simulink model "cvtModel"  (R2019a)
settings: Solver=VariableStepAuto  StartTime=0.0  StopTime=80  FixedStep=1e-3  RelTol=1e-3  AbsTol=1e-3  EnableMultiTasking=on
PreLoadFcn:
  | m1=3.5;
  | m2=3.2;
  | mr1=0.8;
  | mr2=0.7;
  | speedVector=[1508.85099817596;1518.45723596462;1530.44196592720;1537.65262467286;1544.87011816615;1563.98348990289;1583.08660951818;1616.48460379372;1668.91395283447;1709.42350201510;1752.30812599583;1799.96340381967;1847.59134265301;1904.74008492967;1971.45405650923;2028.61646828115;2083.40038787914;2140.55254752961;2190.54189166781;2259.62068592604;2323.95274795787;2376.37867962481;2443.06531221387;2519.28983511532;2576.50350749443;2612.24923757958;2650.37004246484;2681.37245769738;2717.13869202541;2771.92602899721;2819.56080257817;2855.26894155137;2890.95315890788;2938.61868885316;2976.76341535511;2991.07537688442;3019.63778721441;3045.79436637996;3071.94069342408;3093.34370561560;3114.80823053575;3141.04340929901;3172.04240715774;3186.35436868705;3214.89627477416;3231.51496362732;3267.18209411476;3333.83797033950;3371.93485360807;3421.93444986770;3488.60057821388;3540.98550139507;3586.19052219491;3617.10408570831;3674.22548899447;3712.24719003915;3731.22044944954;3740.69340965949;3759.66325169607;3771.50786933232;3785.72414439486;3792.79810818800;3797.48674505959;3802.17879930499;3806.87085355039;3816.26521416264;3820.89917305322;3827.93896310823;3835.00950952755;3839.71865064202];
  | torqueVector=[15.4893802008608;16.0795925394548;16.6441434720229;17.1317101865136;17.6705997130559;18.1068436154950;18.4661032998565;18.8510243902439;19.0563156384505;19.1846226685796;19.2616068866571;19.3899139167862;19.3129296987087;19.1846226685796;19.3385911047346;19.3129296987087;19.3129296987087;19.2102840746054;18.9793314203730;19.0049928263988;19.1589612625538;19.3385911047346;19.2872682926829;19.3129296987087;19.6721893830703;19.8004964131994;19.8774806312769;20.1597560975610;20.4420315638450;20.4676929698709;20.4420315638450;20.2880631276901;19.9544648493544;20.1597560975610;20.4163701578192;20.5703385939742;20.4163701578192;20.0827718794835;19.6721893830703;19.4155753228120;19.6208665710186;19.8774806312769;20.1340946915351;20.2880631276901;19.9801262553802;19.5695437589670;19.1076384505021;18.8253629842181;18.7227173601148;18.5687489239598;18.3634576757532;18.2351506456241;17.8502295552367;17.4653084648493;17.1317101865136;16.4645136298422;15.8486398852224;15.4380573888092;14.7965222381636;14.3089555236729;13.7444045911047;13.2055150645624;12.6409641319943;12.1020746054519;11.5631850789096;10.5623902439024;9.58725681492108;8.79175322812051;8.22720229555236;7.81661979913916];
model workspace (MAT data in the model file):
  DOWN_TABLE = [0  5  20  35; 0  5  20  35; 0  5  25  40; 0  5  30  50; 0  30  50  80; 0  30  50  80]
  DOWN_TH_BP = [0; 0.05; 0.4; 0.5; 0.9; 1]
  TWAIT = 2
  UP_TABLE = [10  30  50  1000000; 10  30  50  1000000; 15  30  50  1000000; 23  41  60  1000000; 40  70  100  1000000; 40  70  100  1000000]
  UP_TH_BP = [0; 0.25; 0.35; 0.5; 0.9; 1]
  clutchRise = 0.1
  eff_tor_rad = 0.4
  engagement_area = 0.0025
  fric_coeff = 0.5
  num_fric_surf = 6
  p0 = 2000000
  peak_normal = 0.55
  pressThresh = 0.05
  velTol = 0.001
undefined symbols (not defined in the file): sigbuilder_block
libraries: fl_lib x21, sdl_lib x9, nesl_utility x8
CloseFcn:
  | try,close(h1_sdl_car),end
  | clear h1_sdl_car
  | 
  | clear simlog_sdl_car
  | clear logsout_sdl_car
Description:
  | Vehicle with Four-Speed Transmission
  | 
  | Copyright 2008-2016 The MathWorks, Inc.
settings Model: FPTRunName=Active  PacingRate=5  ExtModeAutoUpdateStatusClock=off  Creator=MathWorks
settings SolverCC: AutoScaleAbsTol=off  ZcThreshold=0  ZeroCrossAlgorithm=Adaptive
settings DataIOCC: LimitDataPoints=on  MaxDataPoints=10000  SaveOutput=off  DSMLogging=off  SaveTime=off  ReturnWorkspaceOutputs=off  SignalLoggingName=logsout_cvtModel
settings OptimizationCC: ExpressionDepthLimit=2147483647  InitFltsAndDblsToZero=on  LifeSpan=inf
settings DebuggingCC: AlgebraicLoopMsg=none  SaveWithParameterizedLinksMsg=none  UnderspecifiedInitializationDetection=Classic  MergeDetectMultiDrivingBlocksExec=none  CheckExecutionContextPreStartOutputMsg=on  SignalResolutionControl=TryResolveAllWithWarning  MaskedZcDiagnostic=none  MultiTaskDSMMsg=warning  MultiTaskCondExecSysMsg=none  SigSpecEnsureSampleTimeMsg=none  FcnCallInpInsideContextMsg=warning  AllowSymbolicDim=off  StateNameClashWarn=warning  SFUnexpectedBacktrackingDiag=warning  SFNoUnconditionalDefaultTransitionDiag=warning  SFExecutionAtInitializationDiag=none  ArithmeticOperatorsInVariantConditions=warning
settings HardwareCC: ProdBitPerPointer=32  ProdBitPerSizeT=32  ProdBitPerPtrDiffT=32  ProdLargestAtomicFloat=None  ProdIntDivRoundTo=Undefined  ProdEndianess=Unspecified  ProdWordSize=32  ProdHWDeviceType=32-bit Generic  TargetBitPerLong=64  TargetBitPerPointer=64  TargetBitPerSizeT=64  TargetBitPerPtrDiffT=64  TargetLongLongMode=on  TargetIntDivRoundTo=Zero  TargetEndianess=LittleEndian  TargetWordSize=64  TargetHWDeviceType=MATLAB Host  ProdEqTarget=off
settings ModelReferenceCC: UpdateModelReferenceTargets=IfOutOfDate  PropagateSignalLabelsOutOfModel=off
settings SFSimCC: SimUseLocalCustomCode=off
settings RTWCC: Description=Generic Real-Time Target  RTWUseLocalCustomCode=off
settings CodeAppCC: StateflowObjectComments=on
settings GRTTargetCC: TargetLangStandard=C89/C90 (ANSI)  CombineOutputUpdateFcns=off  GRTInterface=on
settings ConfigComp: CovMetricSettings=dw  CovSaveCumulativeToWorkspaceVar=on  CovSaveSingleToWorkspaceVar=on  CovExternalEMLEnable=off  CovBoundaryAbsTol=1.0e-5
settings SimscapeCC: SimscapeNormalizeSystem=off  SimscapeLogType=all  SimscapeLogSimulationStatistics=on

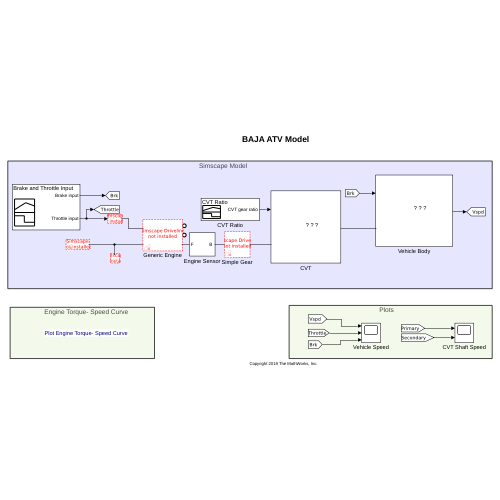
[thumbnail: Simulink's stored preview of the top-level diagram]
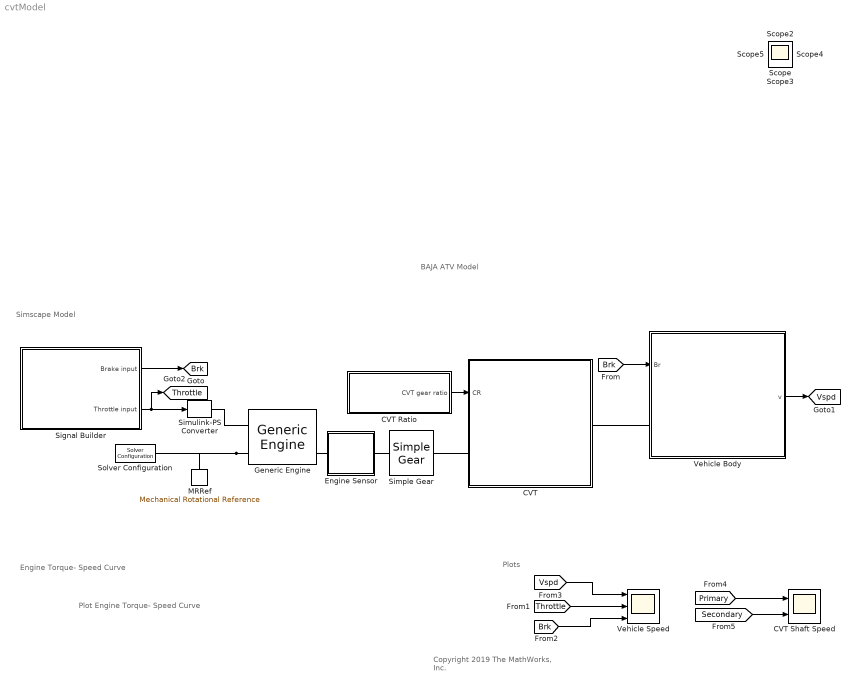
== system cvtModel ==
  note: Simscape Model
  note: Plots
  note: BAJA ATV Model
  note: Copyright 2019 The MathWorks, Inc.
  note: Plot Engine Torque- Speed Curve
  note: Engine Torque- Speed Curve
  CVT : Subsystem
      mask Display: image("CVT.jpg")
  CVT Ratio : Subsystem  Tag=STV Subsys  LoadFcn=sigbuilder_block('load');  StartFcn=sigbuilder_block('start');  StopFcn=sigbuilder_block('stop');  ClipboardFcn=sigbuilder_block('clipboard');  mask(Sigbuilder block){tuvar=[0:10]}
      mask help: Simulink:masks:SigbuilderBlock_MD
      mask init:
      | if ~strcmp(get_param(bdroot(gcbh),'SimulationStatus'),'stopped') tuvar = sigbuilder_block('maskInit'); end
      settings: CopyFcn=sigbuilder_block('copy');  DeleteFcn=sigbuilder_block('delete');  ModelCloseFcn=sigbuilder_block('modelClose');  PreSaveFcn=sigbuilder_block('preSave');  PauseFcn=sigbuilder_block('pause');  ContinueFcn=sigbuilder_block('continue');  NameChangeFcn=sigbuilder_block('namechange');  OpenFcn=sigbuilder_block('open',[6 61.5 948 414.75 ]);  CloseFcn=sigbuilder_block('close');
      mask Display: plot(0, 0, 100, 100,[2, 2, 32, 32, 2], [68, 8, 8, 68, 68],[32, 2], [38, 38], [32, 19, 2],[53, 60, 44], [32, 17, 17, 2],[16, 16, 31, 31]);txt = getActiveGroup(gcbh);text(2, 100, txt,'verticalAlignment', 'top');
  CVT Shaft Speed : Scope  NumInputPorts=2
  Engine Sensor : Subsystem
  Generic Engine : sdl_lib/Engines/Generic Engine  model_parameterization=2  engine_type=1  P_max=100 kW  w_P_max=4500 rpm  w_max=5000 rpm  w_min=500 rpm  w_tab=speedVector rpm  trq_tab=torqueVector N*m  pwr_tab=[20, 40, 78, 120, 145, 148, 125, 60] kW  interp_method=simscape.enum.interpolation.linear  model_inertia=1  inertia=1 kg*m^2  initial_velocity=2100 rpm  model_time_constant=0  time_constant=0.4 s  T0=0  w_thr=100 rpm  idle_speed=0  idle_speed_reference=2500 rpm  tau_controller=1 s  idle_w_thr=1 rpm  redline=0  redline_speed=5000 rpm  tau_redline=1 s  redline_w_thr=1 rpm  fc_model=0  fc_per_rev=25 mg/rev  displaced_volume=400 cm^3  rev_per_cycle=2  fc_w_tab=[1000, 2000, 3000, 4000, 5000, 6000] rpm  fc_trq_tab=[0, 80, 160, 200, 240, 320, 360, 400] N*m  fc_tab=[.5, .9, 1.4, 1.6, 1.9, 2.7, 3.4, 4.4; 1, 1.7, 2.7, 3.1, 3.6, 5, 6, 7.4; 1.4, 2.7, 4, 4.8, 5.6, 7.5, 8.5, 10.5; 2, 3.6, 5.8, 6.7, 8, 10.4, 11.7, 13.3; 2.5, 4.8, 7.9, 9.4, 10.8, 14, 16.2, 18.6; 3.1, 6, 10.3, 11.9, 13.8, 18.4, 22, 26.5] g/s  bmep_tab=[0, 250, 500, 625, 750, 1000, 1150, 1250] kPa  bsfc_tab=[410, 380, 300, 280, 270, 290, 320, 380; 410, 370, 290, 270, 260, 270, 285, 320; 415, 380, 290, 275, 265, 270, 270, 300; 420, 390, 310, 290, 285, 280, 280, 285; 430, 410, 340, 320, 310, 300, 310, 320; 450, 430, 370, 340, 330, 330, 350, 380] g/hr/kW  fc_interp_method=simscape.enum.interpolation.linear
      settings: SourceProductName=Simscape Driveline
  MRRef : fl_lib/Mechanical/Rotational Elements/Mechanical Rotational Reference
  Signal Builder : Subsystem  Tag=STV Subsys  LoadFcn=sigbuilder_block('load');  StartFcn=sigbuilder_block('start');  StopFcn=sigbuilder_block('stop');  ClipboardFcn=sigbuilder_block('clipboard');  mask(Sigbuilder block){tuvar=[0:10]}
      mask help: Simulink:masks:SigbuilderBlock_MD
      mask init:
      | if ~strcmp(get_param(bdroot(gcbh),'SimulationStatus'),'stopped') tuvar = sigbuilder_block('maskInit'); end
      settings: CopyFcn=sigbuilder_block('copy');  DeleteFcn=sigbuilder_block('delete');  ModelCloseFcn=sigbuilder_block('modelClose');  PreSaveFcn=sigbuilder_block('preSave');  PauseFcn=sigbuilder_block('pause');  ContinueFcn=sigbuilder_block('continue');  NameChangeFcn=sigbuilder_block('namechange');  OpenFcn=sigbuilder_block('open',[235.5 66.5 481 367 ]);  CloseFcn=sigbuilder_block('close');
      mask Display: plot(0, 0, 100, 100,[2, 2, 32, 32, 2], [68, 8, 8, 68, 68],[32, 2], [38, 38], [32, 19, 2],[53, 60, 44], [32, 17, 17, 2],[16, 16, 31, 31]);txt = getActiveGroup(gcbh);text(2, 100, txt,'verticalAlignment', 'top');
  Simple Gear : sdl_lib/Gears/Simple Gear  ratio=4  rotation_direction=1  friction_model=1  T_noload=0.1 N*m  T_nom=5 N*m  efficiency_nom=0.8  efficiency=0.8  mu_visc=[0, 0] N*m/(rad/s)  w_thr=0.01 rad/s  pwr_thr=0.001 W  enable_faults=0  efficiency_fault=0.05  external_fault=simscape.enum.onoff.off  temporal_fault=0  fault_time=5 s  fault_angles=pi / 12 rad  report_fault=1  temperature_TLU=[280, 300, 320] K  load_TLU=[1, 5, 10] N*m  efficiency_TLU=[.95, .9, .85]  efficiency_TLU2=[.85, .8, .75; .95, .9, .85; .85, .8, .7]  thermal_mass=50 J/K  T_init=300 K
      settings: SourceProductName=Simscape Driveline
  Simulink-PS Converter : nesl_utility/Simulink-PS Converter  PhysicalDomain=network_engine_domain  SubClassName=ps_input  LeftPortType=input  RightPortType=output  PseudoPeriodic=off  Frequencies=[]  NoiseDistribution=none  NoiseParameters=[]  Unit=1  AffineConversion=off  FilteringAndDerivatives=zero  SimscapeFilterOrder=1  InputFilterTimeConstant=0.001  UdotUserProvided=1
  Solver Configuration : nesl_utility/Solver Configuration  PhysicalDomain=network_engine_domain  SubClassName=solver  LeftPortType=input  RightPortType=generic  Tones=[]  Harmonics=[]  SimulateNoise=off  Profile=off  UseLocalSampling=off  EnableSwitchedLinearOptims=on  FrequencyDomain=off  UseCCode=off  RelTol=0.001  AbsTol=1e-06  MinStep=1e-09  ToWorkspace=off  RevertToSquareIcSolve=off  NumHomotopyIterations=100  PhasorMode=off  PhasorModeNumHarmonics=1  DoDC=off  ResidualTolerance=1e-9  UseLocalSolver=off  LocalSolverChoice=NE_BACKWARD_EULER_ADVANCER  LocalSolverSampleTime=0.001  DoFixedCost=off  MaxNonlinIter=3  MaxModeIter=2  LinearAlgebra=Sparse  EquationFormulation=NE_TIME_EF  DelaysMemoryBudget=1024  AutomaticFiltering=on  FilteringTimeConstant=0.001  PartitionStorageMethod=AS_NEEDED  PartitionMemoryBudget=1024
  Vehicle Body : Subsystem  Tag=PublishSubsystem
      mask Display: image("vehicleBody.jpg")
  Vehicle Speed : Scope  NumInputPorts=3
  Scope{,2..5} (5 alike) : Scope
  tag scope: Brk=global, Throttle=global, Vspd=global
  wires:
  Signal Builder/1(Brake input) -> [Brk]
  [Primary] -> CVT Shaft Speed/1
  [Brk] -> Vehicle Body/1(Br)
  [Throttle] -> Vehicle Speed/2
  [Vspd] -> Vehicle Speed/1
  Vehicle Body/1(v) -> [Vspd]
  CVT Ratio/1(CVT gear ratio) -> CVT/1(CR)
  [Brk] -> Vehicle Speed/3
  [Secondary] -> CVT Shaft Speed/2
  Signal Builder/2(Throttle input) -> Simulink-PS Converter/1, [Throttle]
  connections:
  Vehicle Body/LConn1 -- CVT/RConn1
  Generic Engine/LConn2 -- MRRef/LConn1 -- Solver Configuration/RConn1
  Generic Engine/RConn3 -- Engine Sensor/LConn1
  Simple Gear/LConn1 -- Engine Sensor/RConn1
  Generic Engine/LConn1 -- Simulink-PS Converter/RConn1
  CVT/LConn1 -- Simple Gear/RConn1

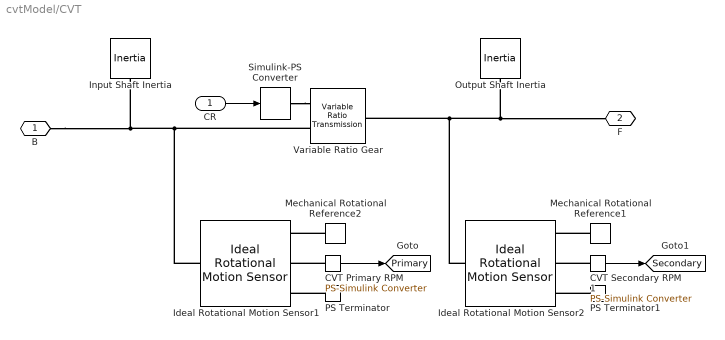
== system cvtModel/CVT ==
  CR : Inport
  "CVT Primary RPM " : nesl_utility/PS-Simulink Converter  PhysicalDomain=network_engine_domain  SubClassName=ps_output  LeftPortType=input  RightPortType=output  PseudoPeriodic=off  Frequencies=[]  Unit=rpm  AffineConversion=off
  CVT Secondary RPM 1 : nesl_utility/PS-Simulink Converter  PhysicalDomain=network_engine_domain  SubClassName=ps_output  LeftPortType=input  RightPortType=output  PseudoPeriodic=off  Frequencies=[]  Unit=rpm  AffineConversion=off
  Ideal Rotational Motion Sensor1 : fl_lib/Mechanical/Mechanical Sensors/Ideal Rotational Motion Sensor  offset=0 rad
  Ideal Rotational Motion Sensor2 : fl_lib/Mechanical/Mechanical Sensors/Ideal Rotational Motion Sensor  offset=0 rad
  Input Shaft Inertia : fl_lib/Mechanical/Rotational Elements/Inertia  inertia=m1*(((18.6e-2)/2)^2+((2.5e-2)/2)^2)/2 kg*m^2  w_specify=on  w_priority=None  w=2500 rpm  w_nominal_specify=off  w_nominal_unit=rad/s  w_nominal_value=1  t_specify=off  t_priority=High  t=0 N*m  t_nominal_specify=off  t_nominal_unit=N*m  t_nominal_value=1
  Mechanical Rotational Reference1 : fl_lib/Mechanical/Rotational Elements/Mechanical Rotational Reference
  Mechanical Rotational Reference2 : fl_lib/Mechanical/Rotational Elements/Mechanical Rotational Reference
  Output Shaft Inertia : fl_lib/Mechanical/Rotational Elements/Inertia  inertia=m2*(((19.8e-2)/2)^2+((1.9e-2)/2)^2)/2 kg*m^2  w_specify=on  w_priority=High  w=0 rpm  w_nominal_specify=off  w_nominal_unit=rad/s  w_nominal_value=1  t_specify=off  t_priority=High  t=0 N*m  t_nominal_specify=off  t_nominal_unit=N*m  t_nominal_value=1
  PS Terminator : fl_lib/Physical Signals/Sinks/PS Terminator
      settings: SourceProductName=Simscape
  PS Terminator1 : fl_lib/Physical Signals/Sinks/PS Terminator
      settings: SourceProductName=Simscape
  Simulink-PS Converter : nesl_utility/Simulink-PS Converter  PhysicalDomain=network_engine_domain  SubClassName=ps_input  LeftPortType=input  RightPortType=output  PseudoPeriodic=off  Frequencies=[]  NoiseDistribution=none  NoiseParameters=[]  Unit=1  AffineConversion=off  FilteringAndDerivatives=zero  SimscapeFilterOrder=1  InputFilterTimeConstant=.001  UdotUserProvided=0
  Variable Ratio Gear : sdl_lib/Couplings & Drives/Variable Ratio Transmission  rotation_direction=1  kp=1e3 N*m/rad  kv=10 N*m/(rad/s)  initial_torque=0 N*m  losses_model=1  efficiency=0.8  mu_visc=[ 0 0 ] N*m/(rad/s)  w_thr=0.01 rad/s  R_specify=off  R_priority=None  R=1  R_nominal_specify=off  R_nominal_unit=1  R_nominal_value=1
      settings: SourceProductName=Simscape Driveline
  B : PMIOPort  Side=Left
  F : PMIOPort  Port=2  Side=Right
  tag scope: Primary=global, Secondary=global
  wires:
  CR/1 -> Simulink-PS Converter/1
  "CVT Primary RPM "/1 -> [Primary]
  CVT Secondary RPM 1/1 -> [Secondary]
  connections:
  Simulink-PS Converter/RConn1 -- Variable Ratio Gear/LConn1
  Variable Ratio Gear/LConn2 -- Ideal Rotational Motion Sensor1/LConn1 -- B/RConn1 -- Input Shaft Inertia/LConn1
  Output Shaft Inertia/LConn1 -- Variable Ratio Gear/RConn1 -- Ideal Rotational Motion Sensor2/LConn1 -- F/RConn1
  "CVT Primary RPM "/LConn1 -- Ideal Rotational Motion Sensor1/RConn2
  PS Terminator/LConn1 -- Ideal Rotational Motion Sensor1/RConn3
  Mechanical Rotational Reference2/LConn1 -- Ideal Rotational Motion Sensor1/RConn1
  PS Terminator1/LConn1 -- Ideal Rotational Motion Sensor2/RConn3
  Mechanical Rotational Reference1/LConn1 -- Ideal Rotational Motion Sensor2/RConn1
  CVT Secondary RPM 1/LConn1 -- Ideal Rotational Motion Sensor2/RConn2

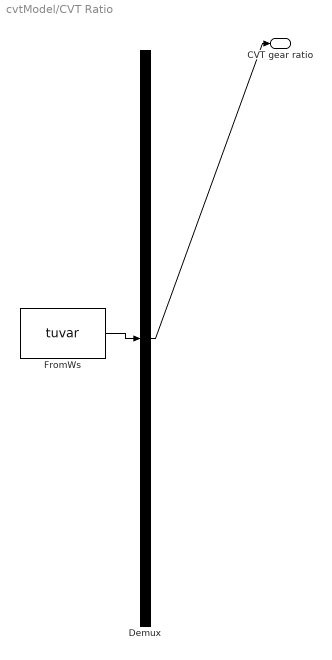
== system cvtModel/CVT Ratio ==
  Demux : Demux  Tag=STV Demux  Outputs=1
      settings: DisplayOption=none
  FromWs : FromWorkspace  Tag=STV FromWs  VariableName=tuvar
      SigBuilderData=|
      | common.afterFinalStr = 'Extrapolate'
      | common.sampleTime = 0
      | dataSet.timeRange = [0 80]
      | dataSet.name = 'CVT Ratio'
      | sbobj.Groups.Name = 'CVT Ratio'
      | sbobj.Groups.Signals.Name = 'CVT gear ratio'
      | sbobj.Groups.Signals.XData = [0 4 35 80]
      | sbobj.Groups.Signals.YData = [2.3 2.3 1.8 1.8]
      | sbobj.Groups.TimeRange = [0 80]
  CVT gear ratio : Outport  Tag=STV Outport  VectorParamsAs1DForOutWhenUnconnected=off
  wires:
  FromWs/1 -> Demux/1
  Demux/1 -> CVT gear ratio/1

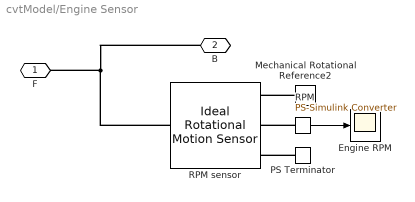
== system cvtModel/Engine Sensor ==
  "    RPM" : nesl_utility/PS-Simulink Converter  PhysicalDomain=network_engine_domain  SubClassName=ps_output  LeftPortType=input  RightPortType=output  PseudoPeriodic=off  Frequencies=[]  Unit=rpm  AffineConversion=off
  "Engine RPM " : Scope
  Mechanical Rotational Reference2 : fl_lib/Mechanical/Rotational Elements/Mechanical Rotational Reference
  PS Terminator : fl_lib/Physical Signals/Sinks/PS Terminator
      settings: SourceProductName=Simscape
  RPM sensor : fl_lib/Mechanical/Mechanical Sensors/Ideal Rotational Motion Sensor  offset=0 rad
  F : PMIOPort  Side=Left
  "B " : PMIOPort  Port=2  Side=Right
  wires:
  "    RPM"/1 -> "Engine RPM "/1
  connections:
  RPM sensor/LConn1 -- "B "/RConn1 -- F/RConn1
  PS Terminator/LConn1 -- RPM sensor/RConn3
  Mechanical Rotational Reference2/LConn1 -- RPM sensor/RConn1
  "    RPM"/LConn1 -- RPM sensor/RConn2

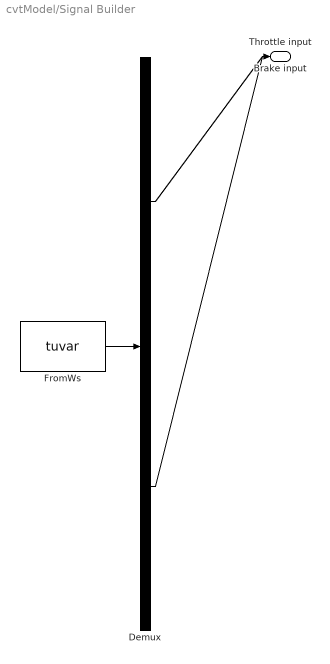
== system cvtModel/Signal Builder ==
  Demux : Demux  Tag=STV Demux  Outputs=2
      settings: DisplayOption=none
  FromWs : FromWorkspace  Tag=STV FromWs  VariableName=tuvar
      SigBuilderData=|
      | common.afterFinalStr = 'Extrapolate'
      | common.sampleTime = 0
      | dataSet.timeRange = [0 80]
      | dataSet.name = 'Brake and Throttle Input'
      | sbobj.Groups.Name = 'Brake and Throttle Input'
      | sbobj.Groups.Signals(1).Name = 'Brake input'
      | sbobj.Groups.Signals(1).XData = [0 80]
      | sbobj.Groups.Signals(1).YData = [0 0]
      | sbobj.Groups.Signals(2).Name = 'Throttle input'
      | sbobj.Groups.Signals(2).XData = [0 20 20 80]
      | sbobj.Groups.Signals(2).YData = [0.3 0.3 1 1]
      | sbobj.Groups.TimeRange = [0 80]
  Brake input : Outport  Tag=STV Outport  VectorParamsAs1DForOutWhenUnconnected=off
  Throttle input : Outport  Tag=STV Outport  Port=2  VectorParamsAs1DForOutWhenUnconnected=off
  wires:
  FromWs/1 -> Demux/1
  Demux/1 -> Brake input/1
  Demux/2 -> Throttle input/1

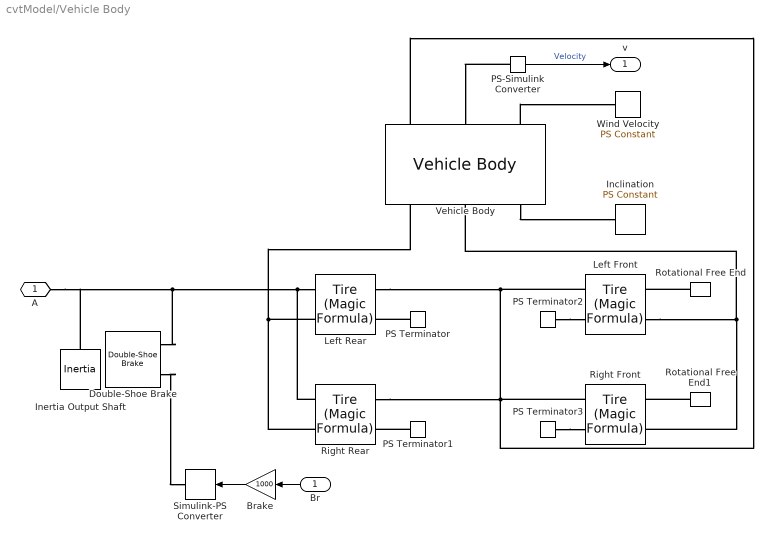
== system cvtModel/Vehicle Body ==
  Br : Inport
  Brake : Gain  Gain=1000
  Double-Shoe Brake : sdl_lib/Brakes & Detents/Rotational/Double-Shoe Brake  r_drum=150 mm  r_act=100 mm  r_pin=125 mm  theta_pin=15 deg  theta_0=5 deg  theta_shoe=120 deg  mu_visc=.01 N*m/(rad/s)  mu=0.3  w_thr=0.01 rad/s  temperature_TLU=[280.0, 300.0, 320.0] K  mu_TLU=[0.1, 0.05, 0.03]  thermal_mass=50 kJ/K  temperature_specify=off  temperature_priority=High  temperature=300 K  temperature_nominal_specify=off  temperature_nominal_unit=K  temperature_nominal_value=1
      settings: SourceProductName=Simscape Driveline
  Inclination : fl_lib/Physical Signals/Sources/PS Constant  constant=0
  Inertia Output Shaft : fl_lib/Mechanical/Rotational Elements/Inertia  inertia=1e-1 kg*m^2  w_specify=on  w_priority=High  w=0 rpm  w_nominal_specify=off  w_nominal_unit=rad/s  w_nominal_value=1  t_specify=off  t_priority=High  t=0 N*m  t_nominal_specify=off  t_nominal_unit=N*m  t_nominal_value=1
  Left Front : sdl_lib/Tires & Vehicles/Tire (Magic Formula)  parameterization=2  F_z1=3000 N  F_x1=3500 N  kappa1=10  B_m=10  C_m=1.9  D_m=1  E_m=0.97  fz0=4000 N  p_Cx=1.685  p_Dx=[1.21, -.037]  p_Ex=[.344, .095, -.02, 0]  p_Kx=[21.51, -.163, .245]  p_Hx=[-.002, .002]  p_Vx=[0, 0]  v_tr_thr=0.1 m/s  r_e=.2794 m  model_compliance=0  stiffness=1e6 N/m  damping=1000 N/(m/s)  model_inertia=1  inertia=1e-2 kg*m^2  initial_velocity=0 rpm  model_resistance=0  resistance_model=1  coeff=0.015  p_tire=250e3 Pa  alpha=-0.003  beta=0.97  coeff_a=84e-4  coeff_b=6.2e-4 s/m  coeff_c=1.6e-4 s^2/m^2  v_thr=0.001 m/s
      settings: SourceProductName=Simscape Driveline
  Left Rear : sdl_lib/Tires & Vehicles/Tire (Magic Formula)  parameterization=2  F_z1=3000 N  F_x1=3500 N  kappa1=10  B_m=10  C_m=1.9  D_m=1  E_m=0.97  fz0=4000 N  p_Cx=1.685  p_Dx=[1.21, -.037]  p_Ex=[.344, .095, -.02, 0]  p_Kx=[21.51, -.163, .245]  p_Hx=[-.002, .002]  p_Vx=[0, 0]  v_tr_thr=0.1 m/s  r_e=.2794 m  model_compliance=0  stiffness=1e6 N/m  damping=1000 N/(m/s)  model_inertia=1  inertia=1e-2 kg*m^2  initial_velocity=0 rpm  model_resistance=1  resistance_model=1  coeff=0.015  p_tire=250e3 Pa  alpha=-0.003  beta=0.97  coeff_a=84e-4  coeff_b=6.2e-4 s/m  coeff_c=1.6e-4 s^2/m^2  v_thr=0.001 m/s
      settings: SourceProductName=Simscape Driveline
  PS Terminator{,1..3} (4 alike) : fl_lib/Physical Signals/Sinks/PS Terminator
      settings: SourceProductName=Simscape
  PS-Simulink Converter : nesl_utility/PS-Simulink Converter  PhysicalDomain=network_engine_domain  SubClassName=ps_output  LeftPortType=input  RightPortType=output  PseudoPeriodic=off  Frequencies=[]  Unit=km/hr  AffineConversion=off
  Right Front : sdl_lib/Tires & Vehicles/Tire (Magic Formula)  parameterization=2  F_z1=3000 N  F_x1=3500 N  kappa1=10  B_m=10  C_m=1.9  D_m=1  E_m=0.97  fz0=4000 N  p_Cx=1.685  p_Dx=[1.21, -.037]  p_Ex=[.344, .095, -.02, 0]  p_Kx=[21.51, -.163, .245]  p_Hx=[-.002, .002]  p_Vx=[0, 0]  v_tr_thr=0.1 m/s  r_e=.2794 m  model_compliance=0  stiffness=1e6 N/m  damping=1000 N/(m/s)  model_inertia=1  inertia=1e-2 kg*m^2  initial_velocity=0 rpm  model_resistance=0  resistance_model=1  coeff=0.015  p_tire=250e3 Pa  alpha=-0.003  beta=0.97  coeff_a=84e-4  coeff_b=6.2e-4 s/m  coeff_c=1.6e-4 s^2/m^2  v_thr=0.001 m/s
      settings: SourceProductName=Simscape Driveline
  Right Rear : sdl_lib/Tires & Vehicles/Tire (Magic Formula)  parameterization=2  F_z1=3000 N  F_x1=3500 N  kappa1=10  B_m=10  C_m=1.9  D_m=1  E_m=0.97  fz0=4000 N  p_Cx=1.685  p_Dx=[1.21, -.037]  p_Ex=[.344, .095, -.02, 0]  p_Kx=[21.51, -.163, .245]  p_Hx=[-.002, .002]  p_Vx=[0, 0]  v_tr_thr=0.1 m/s  r_e=.2794 m  model_compliance=0  stiffness=1e6 N/m  damping=1000 N/(m/s)  model_inertia=1  inertia=1e-2 kg*m^2  initial_velocity=0 rpm  model_resistance=0  resistance_model=1  coeff=0.015  p_tire=250e3 Pa  alpha=-0.003  beta=0.97  coeff_a=84e-4  coeff_b=6.2e-4 s/m  coeff_c=1.6e-4 s^2/m^2  v_thr=0.001 m/s
      settings: SourceProductName=Simscape Driveline
  Rotational Free End : fl_lib/Mechanical/Rotational Elements/Rotational Free End  w_specify=off  w_priority=None  w=0 rad/s  w_nominal_specify=off  w_nominal_unit=rad/s  w_nominal_value=1
      settings: SourceProductName=Simscape
  Rotational Free End1 : fl_lib/Mechanical/Rotational Elements/Rotational Free End  w_specify=off  w_priority=None  w=0 rad/s  w_nominal_specify=off  w_nominal_unit=rad/s  w_nominal_value=1
      settings: SourceProductName=Simscape
  Simulink-PS Converter : nesl_utility/Simulink-PS Converter  PhysicalDomain=network_engine_domain  SubClassName=ps_input  LeftPortType=input  RightPortType=output  PseudoPeriodic=off  Frequencies=[]  NoiseDistribution=none  NoiseParameters=[]  Unit=N  AffineConversion=off  FilteringAndDerivatives=zero  SimscapeFilterOrder=1  InputFilterTimeConstant=0.001  UdotUserProvided=1
  Vehicle Body : sdl_lib/Tires & Vehicles/Vehicle Body  mass=250 kg  n_w=2  x_f=1 m  x_r=.35 m  y_c=0.7 m  model_pitch=0  inertia=4000 kg*m^2  suspension_model=1  k_f=1e4 N/m  b_f=1e4 N/(m/s)  k_r=1e4 N/m  b_r=1e4 N/(m/s)  k_f_TLU=[-2000, -1000, 0, 1000, 2000] N  x_f_TLU=[-.4, -.2, 0, .2, .4] m  b_f_TLU=[-200, -100, 0, 100, 200] N  v_f_TLU=[-4, -2, 0, 2, 4] m/s  k_r_TLU=[-2000, -1000, 0, 1000, 2000] N  x_r_TLU=[-.4, -.2, 0, .2, .4] m  b_r_TLU=[-200, -100, 0, 100, 200] N  v_r_TLU=[-4, -2, 0, 2, 4] m/s  interp_method=simscape.enum.interpolation.linear  extrap_method=simscape.enum.extrapolation.linear  model_hardstop=0  upper_bound_f=.25 m  lower_bound_f=-.25 m  stop_k_f=1e6 N/m  stop_b_f=150 N/(m/s)  upper_bound_r=.25 m  lower_bound_r=-.25 m  stop_k_r=1e6 N/m  stop_b_r=150 N/(m/s)  initial_pitch=0 rad  initial_pitch_rate=0 rad/s  g=9.81 m/s^2  liftoff_warning=0  area=.735482 m^2  Cd=1.92  rho=1.18 kg/m^3  v_specify=on  v_priority=High  v=0 m/s  v_nominal_specify=off  v_nominal_unit=m/s  v_nominal_value=1
      settings: SourceProductName=Simscape Driveline
  Wind Velocity : fl_lib/Physical Signals/Sources/PS Constant  constant=0
  A : PMIOPort  Side=Left
  v : Outport  VectorParamsAs1DForOutWhenUnconnected=off
  wires:
  PS-Simulink Converter/1 -> v/1  "Velocity"
  Brake/1 -> Simulink-PS Converter/1
  Br/1 -> Brake/1
  connections:
  Right Rear/LConn1 -- Vehicle Body/RConn1 -- Left Rear/LConn1
  Right Rear/LConn2 -- Inertia Output Shaft/LConn1 -- A/RConn1 -- Double-Shoe Brake/LConn2 -- Left Rear/LConn2
  Right Rear/RConn2 -- Vehicle Body/LConn1 -- Right Front/RConn2 -- Left Rear/RConn2 -- Left Front/RConn2
  Vehicle Body/LConn3 -- Wind Velocity/RConn1
  PS Terminator3/LConn1 -- Right Front/RConn1
  PS Terminator1/LConn1 -- Right Rear/RConn1
  Rotational Free End/LConn1 -- Left Front/LConn2
  PS Terminator2/LConn1 -- Left Front/RConn1
  Left Front/LConn1 -- Right Front/LConn1 -- Vehicle Body/RConn2
  Rotational Free End1/LConn1 -- Right Front/LConn2
  PS Terminator/LConn1 -- Left Rear/RConn1
  PS-Simulink Converter/LConn1 -- Vehicle Body/LConn2
  Vehicle Body/RConn3 -- Inclination/RConn1
  Double-Shoe Brake/LConn1 -- Simulink-PS Converter/RConn1
